simulink library "GOcontroll_Crank"  (R2023b)
settings: Solver=ode45  StartTime=0.0  StopTime=10.0  RelTol=1e-3  EnableMultiTasking=on
PreLoadFcn:
  | compile_crank_mex;
undefined symbols (not defined in the file or in its folder): DiscIntNeverNeededParam, missing
libraries: simulink x2
(part 1 of 2)
settings Model: Creator=HANcoder  LastModifiedBy=maud
settings Model: ModifiedHistory=|
  | la_obwlf -- Thu Sep 01 12:12:55 2016 -- Version 0.33
  | 
  | 
  | 
  | 
  | 
  | 
  | la_obwlf -- Thu Sep 01 09:23:34 2016 -- Version 0.33
  | changed the version in the Base Sample Time block
  | 
  | 
  | 
  | la_obwlf -- Tue Aug 30 15:48:17 2016 -- Version 0.33
settings SolverCC: AlgebraicLoopSolver=TrustRegion
settings DataIOCC: LimitDataPoints=on  SaveFormat=Array  SignalLoggingSaveFormat=ModelDataLogs  ReturnWorkspaceOutputs=off
settings OptimizationCC: ExpressionDepthLimit=2147483647  LifeSpan=inf
settings DebuggingCC: UnderspecifiedInitializationDetection=Classic  MergeDetectMultiDrivingBlocksExec=none  SolverPrmCheckMsg=warning  FcnCallInpInsideContextMsg=warning  UnconnectedInputMsg=warning  UnconnectedOutputMsg=warning  UnconnectedLineMsg=warning  StateNameClashWarn=warning  SFUnexpectedBacktrackingDiag=warning  SFNoUnconditionalDefaultTransitionDiag=warning  SFExecutionAtInitializationDiag=none  ArithmeticOperatorsInVariantConditions=warning
settings HardwareCC: ProdBitPerPointer=32  ProdBitPerSizeT=32  ProdBitPerPtrDiffT=32  ProdLargestAtomicFloat=None  ProdIntDivRoundTo=Undefined  ProdEndianess=Unspecified  ProdWordSize=32  ProdHWDeviceType=32-bit Generic
settings ModelReferenceCC: EnableRefExpFcnMdlSchedulingChecks=on  PropagateSignalLabelsOutOfModel=off
settings SFSimCC: SimUseLocalCustomCode=off  CustomCodeUndefinedFunction=UseInterfaceOnly
settings RTWCC: RTWUseLocalCustomCode=off
settings CodeAppCC: StateflowObjectComments=on
settings GRTTargetCC: TargetLangStandard=C89/C90 (ANSI)  CombineOutputUpdateFcns=off  GRTInterface=on
settings ConfigComp: CovMetricSettings=dw  CovSaveCumulativeToWorkspaceVar=on  CovSaveSingleToWorkspaceVar=on  CovExternalEMLEnable=off  CovSFcnEnable=off

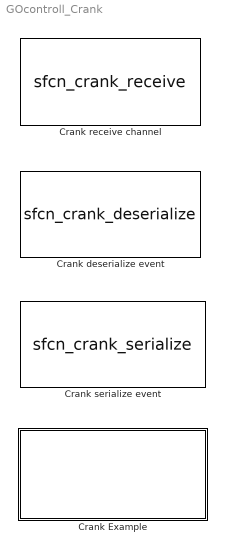
== system GOcontroll_Crank ==
  Crank Example : Subsystem
  Crank deserialize event : S-Function  FunctionName=sfcn_crank_deserialize  Parameters=channel,event_num,event_name,output_names,output_datatypes  SFunctionDeploymentMode=off  EnableBusSupport=off  mask(Crank deserialize event){channel="", event_name=event, event_num="", output_names=[], output_datatypes=[]}
      mask prompts: event_name "Event to deserialize"
      mask help:
      | Block to deserialize an event coming from a gre_io channel
      |
      | Place this block in a function call subsystem that is called by a Crank receive channel block, then link the event ports of these to blocks.
      | Multiple of this blocks can then be placed in this subsystem and attached to the event line.
      |
      | Select the event from the list to deserialize.
      mask Callback channel:
      | try
      |         graph = sltrace(gcb,"Source",TraceAll="on",BlockPath="on");
      |     catch
      |         return;
      |     end
      |     if isempty(graph.SrcBlocks)
      |         error("Could not find a source Crank receive channel block attached to this one");
      |     end
      |     receive = getBlock(graph.SrcBlocks(1),1);
      |     mask = Simulink.Mask.get(gcb);
      |     pars = mask.Parameters;
      |     set_param(gcb, 'channel', char(get_param(receive,'channel')));
      |     mask.getParameter('event_name').TypeOptions = eval(string(get_param(receive,'events')));
      mask TypeOptions event_name: event
      mask Callback event_name:
      | try
      |         graph = sltrace(gcb,"Source",TraceAll="on",BlockPath="on");
      |     catch
      |         return;
      |     end
      |     if isempty(graph.SrcBlocks)
      |         error("Could not find a source Crank receive channel block attached to this one");
      |     end
      |     receive = getBlock(graph.SrcBlocks(1),1);
      |     mask = Simulink.Mask.get(gcb);
      |     pars = mask.Parameters;
      |     set_param(gcb, 'channel', char(get_param(receive,'channel')));
      |     mask.getParameter('event_name').TypeOptions = eval(string(get_param(receive,'events')));
      |     events = eval(string(get_param(receive, 'events')));
      |     eventname = string(get_param(gcb,'event_name'));
      |     index =  find(strcmp(events,eventname));
      |     set_param(gcb, 'event_num',num2str(max(index-1, 0)));
      |     num_fields = eval(string(get_param(receive, 'num_fields')));
      |     field_types = eval(string(get_param(receive, 'field_types')));
      |     field_names = eval(string(get_param(receive, 'field_names')));
      |     if num_fields(index) > 0
      |         names = sprintf('\"%s\",',field_names(index,1:num_fields(index)));
      |         names = names(1:end-1);
      |         names = sprintf('[%s]',names);
      |         set_param(gcb, 'output_names', names);
      |         set_param(gcb, 'output_datatypes', mat2str(field_types(index,1:num_fields(index))));
      |     else
      |         set_param(gcb, 'output_names', '[]');
      |         set_param(gcb, 'output_datatypes', '[]');
      |     end
      mask Display:
      | fprintf('Crank deserialize event\n%s',event_name);
      | text(2, 6, blockset_crank_version());
      | port_label('input', 1, 'event');
      | port_label('output', 1, 'function call');
      | outputnamesarr = eval(output_names);
      | for idx = 1:length(outputnamesarr)
      |     port_label('output', idx+1, outputnamesarr(idx));
      | end
  Crank receive channel : S-Function  FunctionName=sfcn_crank_receive  Parameters=tsamp,nbuff_len,channel,events,num_events,header  SFunctionDeploymentMode=off  EnableBusSupport=off  mask(Crank receive channel){field_names=string([]), num_fields=double([]), field_types=double([]), fmts=string([]), tsamp=-1, nbuff_len=1, channel='channel', header_text=, events=string([]), header="", num_events=0}
      mask prompts: tsamp "Sample time"; nbuff_len "Crank serialized data buffer size"; channel "Crank channel name"; header_text "Header file"
      mask help:
      | Block to receive events coming through a gre_io channel
      |
      | Press the button to Select a crank header that contains the definitions of all the events on this channel.
      | Set the desired sample time to determine how often to process events
      | Set the buffer size for your gre_io_serialized_data_t buffer
      | Set the receive channel name
      mask init:
      | if ~ischar(channel)
      |         error("The channel name needs to be of type char, enter it between single quotes instead of double ones");
      |     end
      |     if nbuff_len <= 0 || mod(nbuff_len,1) > 0
      |         error("The nbuffer length needs to be a positive integer");
      |     end
      mask DialogControl Control2 Prompt: Select crank header
      mask DialogControl Control2 Callback:
      | mask = Simulink.Mask.get(gcb);
      |     pars = mask.Parameters;
      |     [file, location] = uigetfile('*.h','Get crank header');
      |     if exist(fullfile(location, file), 'file') == 2
      |         header_text = fileread(fullfile(location, file));
      |         events = processCrankHeader(header_text);
      |         set_param(gcb, 'header_text', header_text);
      |         set_param(gcb, 'header', char(sprintf("\'%s\'",file)));
      |         names = sprintf('\"%s\",',events.names);
      |         names = names(1:end-1);
      |         names = sprintf('[%s]',names);
      |         set_param(gcb, 'events', names);
      |         set_param(gcb, 'fmts', mat2str(events.fmts));
      |         set_param(gcb, 'num_fields', mat2str(events.num_fields));
      |         set_param(gcb, 'field_names', mat2str(events.field_names));
      |         set_param(gcb, 'field_types', mat2str(events.field_types));
      |         set_param(gcb, 'num_events', num2str(length(events.names)));
      |     end
      mask Display:
      | fprintf('Crank receive channel\n%s',channel);
      | text(2, 6, blockset_crank_version());
      | port_label('output', 1, 'function call');
      | port_label('output', 2, 'event');
  Crank serialize event : S-Function  FunctionName=sfcn_crank_serialize  Parameters=tsamp,channel,event_name,input_names,input_datatypes,header  SFunctionDeploymentMode=off  EnableBusSupport=off  mask(Crank serialize event){field_types=[], tsamp=-1, channel='channel', event_name=event, input_names=[], input_datatypes=[], header='', header_text=, num_fields=[], field_names=[], fmts=[], events=[]}
      mask prompts: tsamp "Sample time"; channel "Crank channel name"; event_name "Event to serialize"; header_text "Header file"
      mask help:
      | Block to serialize an event and send it through a gre_io channel
      |
      | Set the sample time to set the update rate of the display
      | Set the channel name on which the events are sent
      | Press the button to select a crank header that contains the event definitions
      | Select an event from the now loaded event list
      mask init:
      | if ~ischar(channel)
      |         error("The channel name needs to be of type char, enter it between single quotes instead of double ones");
      |     end
      mask TypeOptions event_name: event
      mask Callback event_name:
      | events = eval(string(get_param(gcb, 'events')));
      |     eventname = char(get_param(gcb,'event_name'));
      |     index =  find(strcmp(events,eventname));
      |     num_fields = eval(string(get_param(gcb, 'num_fields')));
      |     field_types = eval(string(get_param(gcb, 'field_types')));
      |     field_names = eval(string(get_param(gcb, 'field_names')));
      |     if num_fields(index) > 0
      |         names = sprintf('\"%s\",',field_names(index,1:num_fields(index)));
      |         names = names(1:end-1);
      |         names = sprintf('[%s]',names);
      |         set_param(gcb, 'input_names', names);
      |         set_param(gcb, 'input_datatypes', mat2str(field_types(index,1:num_fields(index))));
      |     else
      |         set_param(gcb, 'input_names', '[]');
      |         set_param(gcb, 'input_datatypes', '[]');
      |     end
      mask DialogControl Control2 Prompt: Select crank header
      mask DialogControl Control2 Callback:
      | mask = Simulink.Mask.get(gcb);
      |     pars = mask.Parameters;
      |     [file, location] = uigetfile('*.h','Get crank header');
      |     if exist(fullfile(location, file), 'file') == 2
      |         header_text = fileread(fullfile(location, file));
      |         events = processCrankHeader(header_text);
      |         set_param(gcb, 'header_text', header_text);
      |         set_param(gcb, 'header', char(sprintf("\'%s\'",file)));
      |         mask.getParameter('event_name').TypeOptions = events.names;
      |         set_param(gcb, 'events', mat2str(events.names));
      |         set_param(gcb, 'fmts', mat2str(events.fmts));
      |         set_param(gcb, 'num_fields', mat2str(events.num_fields));
      |         set_param(gcb, 'field_names', mat2str(events.field_names));
      |         set_param(gcb, 'field_types', mat2str(events.field_types));
      |     end
      mask Display:
      | fprintf('Crank serialize event\nChannel: %s\nEvent: %s',channel, event_name);
      | text(2, 6, blockset_crank_version());
      | inputnamesarr = eval(input_names);
      | for idx = 1:length(inputnamesarr)
      |     port_label('input', idx, inputnamesarr(idx));
      | end

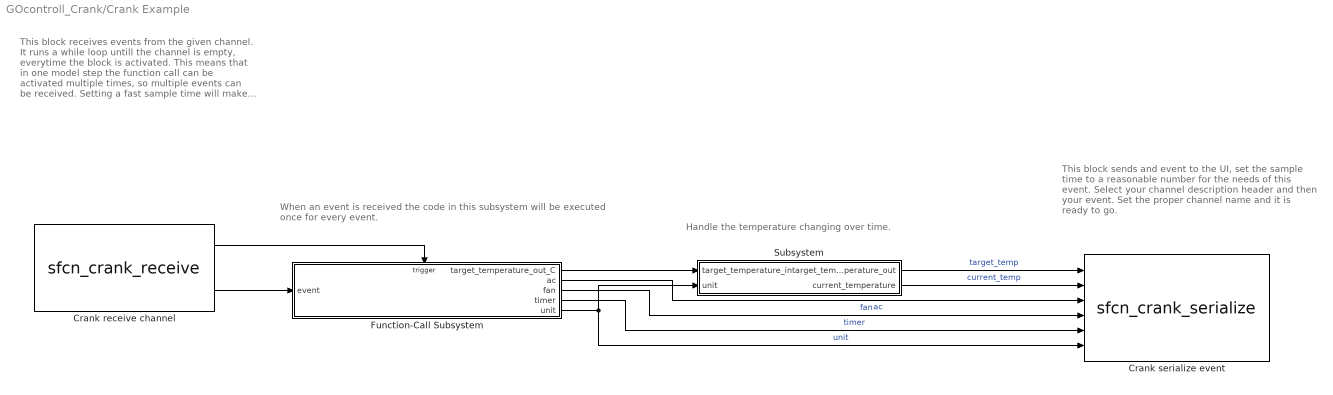
== system GOcontroll_Crank/Crank Example ==
  note: This block sends and event to the UI, set
      | the sample time to a reasonable number
      | for the needs of this event.
      | Select your channel description header
      | and then your event. Set the proper
      | channel name and it is ready to go.
  note: Handle the temperature changing over
      | time.
  note: When an event is received the code in this subsystem
      | will be executed once for every event.
  note: This block receives events from the
      | given channel. It runs a while loop
      | untill the channel is empty, everytime
      | the block is activated.
      | This means that in one model step
      | the function call can be activated
      | multiple times, so multiple events
      | can be received.
      | Setting a fast sample time will make
      | simulink read from the channel more
      | often, giving faster response times but
      | slightly more overhead, though this
      | should not be very significant.
  Crank receive channel : S-Function  AncestorBlock=GOcontroll_Crank/Crank receive channel  FunctionName=sfcn_crank_receive  Parameters=tsamp,nbuff_len,channel,events,num_events,header  SFunctionDeploymentMode=off  EnableBusSupport=off  mask(Crank receive channel){field_names=["num" "unit" string(missing) string(missing) string(missing) string(missing);"num" "unit" string(missing) string(missing) string(missing) string(missing);"target_temperature" "current_temperature" "ac" "fan" "timer" "units"], num_fields=[2 2 6 0 0 0 0], field_types=[5 5 0 0 0 0;5 5 0 0 0 0;4 4 3 3 3 3], fmts=["2u1 num 2u1 unit" "2u1 num 2u1 unit" "2s1 target_temperature 2s1 current_temperature 1u1 ac 1u1 fan 1u1 timer 1u1 units" "" "" "" ""], tsamp=0.01, nbuff_len=100, channel='thermostat_backend', header_text=|, events=["decrease_temperature","increase_temperature","thermostat_update","toggle_ac","toggle_fan","toggle_timer","toggle_units"], header='ThermostatIO_events.h', num_events=7}
      mask header_text=|
      | #define DECREASE_TEMPERATURE_EVENT "decrease_temperature"
      | #define DECREASE_TEMPERATURE_FMT "2u1 num 2u1 unit"
      | typedef struct {
      | 	uint16_t 		num;
      | 	uint16_t 		unit;
      | } decrease_temperature_event_t;
      |
      | #define INCREASE_TEMPERATURE_EVENT "increase_temperature"
      | #define INCREASE_TEMPERATURE_FMT "2u1 num 2u1 unit"
      | typedef struct {
      | 	uint16_t 		num;
      | 	uint16_t 		unit;
      | } increase_temperature_event_t;
      |
      | #define THERMOSTAT_UPDATE_EVENT "thermostat_update"
      | #define THERMOSTAT_UPDATE_FMT "2s1 target_temperature 2s1 current_temperature 1u1 ac 1u1 fan 1u1 timer 1u1 units"
      | typedef struct {
      | 	int16_t 		target_temperature;
      | 	int16_t 		current_temperature;
      | 	uint8_t 		ac;
      | 	uint8_t 		fan;
      | 	uint8_t 		timer;
      | 	uint8_t 		units;
      | } thermostat_update_event_t;
      |
      | #define TOGGLE_AC_EVENT "toggle_ac"
      |
      | #define TOGGLE_FAN_EVENT "toggle_fan"
      |
      | #define TOGGLE_TIMER_EVENT "toggle_timer"
      |
      | #define TOGGLE_UNITS_EVENT "toggle_units"
      mask prompts: tsamp "Sample time"; nbuff_len "Crank serialized data buffer size"; channel "Crank channel name"; header_text "Header file"
      mask help:
      | Block to receive events coming through a gre_io channel
      |
      | Press the button to Select a crank header that contains the definitions of all the events on this channel.
      | Set the desired sample time to determine how often to process events
      | Set the buffer size for your gre_io_serialized_data_t buffer
      | Set the receive channel name
      mask init: same as GOcontroll_Crank/Crank receive channel
      mask DialogControl Control2 Prompt: Select crank header
      mask DialogControl Control2 Callback:
      | mask = Simulink.Mask.get(gcb);
      |     pars = mask.Parameters;
      |     [file, location] = uigetfile('*.h','Get crank header');
      |     if exist(fullfile(location, file), 'file') == 2
      |         header_text = fileread(fullfile(location, file));
      |         events = processCrankHeader(header_text);
      |         set_param(gcb, 'header_text', header_text);
      |         set_param(gcb, 'header', char(sprintf("\'%s\'",file)));
      |         names = sprintf('\"%s\",',events.names);
      |         names = names(1:end-1);
      |         names = sprintf('[%s]',names);
      |         set_param(gcb, 'events', names);
      |         set_param(gcb, 'fmts', mat2str(events.fmts));
      |         set_param(gcb, 'num_fields', mat2str(events.num_fields));
      |         set_param(gcb, 'field_names', mat2str(events.field_names));
      |         set_param(gcb, 'field_types', mat2str(events.field_types));
      |         set_param(gcb, 'num_events', num2str(length(events.names)));
      |     end
      mask Display:
      | fprintf('Crank receive channel\n%s',channel);
      | text(2, 6, blockset_crank_version());
      | port_label('output', 1, 'function call');
      | port_label('output', 2, 'event');
  Crank serialize event : S-Function  AncestorBlock=GOcontroll_Crank/Crank serialize event  FunctionName=sfcn_crank_serialize  Parameters=tsamp,channel,event_name,input_names,input_datatypes,header  SFunctionDeploymentMode=off  EnableBusSupport=off  mask(Crank serialize event){field_types=[5 5 0 0 0 0;5 5 0 0 0 0;4 4 3 3 3 3], tsamp=0.02, channel='thermostat_frontend', event_name=thermostat_update, input_names=["target_temperature","current_temperature","ac","fan","timer","units"], input_datatypes=[4 4 3 3 3 3], header='ThermostatIO_events.h', header_text=|, num_fields=[2 2 6 0 0 0 0], field_names=["num" "unit" string(missing) string(missing) string(missing) string(missing);"num" "unit" string(missing) string(missing) string(missing) string(missing);"target_temperature" "current_temperature" "ac" "fan" "timer" "units"], fmts=["2u1 num 2u1 unit" "2u1 num 2u1 unit" "2s1 target_temperature 2s1 current_temperature 1u1 ac 1u1 fan 1u1 timer 1u1 units" "" "" "" ""], events=["decrease_temperature" "increase_temperature" "thermostat_update" "toggle_ac" "toggle_fan" "toggle_timer" "toggle_units"]}
      mask header_text=|
      | #define DECREASE_TEMPERATURE_EVENT "decrease_temperature"
      | #define DECREASE_TEMPERATURE_FMT "2u1 num 2u1 unit"
      | typedef struct {
      | 	uint16_t 		num;
      | 	uint16_t 		unit;
      | } decrease_temperature_event_t;
      |
      | #define INCREASE_TEMPERATURE_EVENT "increase_temperature"
      | #define INCREASE_TEMPERATURE_FMT "2u1 num 2u1 unit"
      | typedef struct {
      | 	uint16_t 		num;
      | 	uint16_t 		unit;
      | } increase_temperature_event_t;
      |
      | #define THERMOSTAT_UPDATE_EVENT "thermostat_update"
      | #define THERMOSTAT_UPDATE_FMT "2s1 target_temperature 2s1 current_temperature 1u1 ac 1u1 fan 1u1 timer 1u1 units"
      | typedef struct {
      | 	int16_t 		target_temperature;
      | 	int16_t 		current_temperature;
      | 	uint8_t 		ac;
      | 	uint8_t 		fan;
      | 	uint8_t 		timer;
      | 	uint8_t 		units;
      | } thermostat_update_event_t;
      |
      | #define TOGGLE_AC_EVENT "toggle_ac"
      |
      | #define TOGGLE_FAN_EVENT "toggle_fan"
      |
      | #define TOGGLE_TIMER_EVENT "toggle_timer"
      |
      | #define TOGGLE_UNITS_EVENT "toggle_units"
      mask prompts: tsamp "Sample time"; channel "Crank channel name"; event_name "Event to serialize"; header_text "Header file"
      mask help:
      | Block to serialize an event and send it through a gre_io channel
      |
      | Set the sample time to set the update rate of the display
      | Set the channel name on which the events are sent
      | Press the button to select a crank header that contains the event definitions
      | Select an event from the now loaded event list
      mask init:
      | if ~ischar(channel)
      |         error("The channel name needs to be of type char, enter it between single quotes instead of double ones");
      |     end
      mask TypeOptions event_name: event
      mask Callback event_name:
      | events = eval(string(get_param(gcb, 'events')));
      |     eventname = char(get_param(gcb,'event_name'));
      |     index =  find(strcmp(events,eventname));
      |     num_fields = eval(string(get_param(gcb, 'num_fields')));
      |     field_types = eval(string(get_param(gcb, 'field_types')));
      |     field_names = eval(string(get_param(gcb, 'field_names')));
      |     if num_fields(index) > 0
      |         names = sprintf('\"%s\",',field_names(index,1:num_fields(index)));
      |         names = names(1:end-1);
      |         names = sprintf('[%s]',names);
      |         set_param(gcb, 'input_names', names);
      |         set_param(gcb, 'input_datatypes', mat2str(field_types(index,1:num_fields(index))));
      |     else
      |         set_param(gcb, 'input_names', '[]');
      |         set_param(gcb, 'input_datatypes', '[]');
      |     end
      mask DialogControl Control2 Prompt: Select crank header
      mask DialogControl Control2 Callback:
      | mask = Simulink.Mask.get(gcb);
      |     pars = mask.Parameters;
      |     [file, location] = uigetfile('*.h','Get crank header');
      |     if exist(fullfile(location, file), 'file') == 2
      |         header_text = fileread(fullfile(location, file));
      |         events = processCrankHeader(header_text);
      |         set_param(gcb, 'header_text', header_text);
      |         set_param(gcb, 'header', char(sprintf("\'%s\'",file)));
      |         mask.getParameter('event_name').TypeOptions = events.names;
      |         set_param(gcb, 'events', mat2str(events.names));
      |         set_param(gcb, 'fmts', mat2str(events.fmts));
      |         set_param(gcb, 'num_fields', mat2str(events.num_fields));
      |         set_param(gcb, 'field_names', mat2str(events.field_names));
      |         set_param(gcb, 'field_types', mat2str(events.field_types));
      |     end
      mask Display:
      | fprintf('Crank serialize event\nChannel: %s\nEvent: %s',channel, event_name);
      | text(2, 6, blockset_crank_version());
      | inputnamesarr = eval(input_names);
      | for idx = 1:length(inputnamesarr)
      |     port_label('input', idx, inputnamesarr(idx));
      | end
  Function-Call Subsystem : Subsystem  TreatAsAtomicUnit=on
  Subsystem : Subsystem
  wires:
  Subsystem/1(target_temperature_out) -> Crank serialize event/1  "target_temp"
  Function-Call Subsystem/1(target_temperature_out_C) -> Subsystem/1(target_temperature_in)
  Subsystem/2(current_temperature) -> Crank serialize event/2  "current_temp"
  Function-Call Subsystem/5(unit) -> Crank serialize event/6, Subsystem/2(unit)  "unit"
  Function-Call Subsystem/4(timer) -> Crank serialize event/5  "timer"
  Function-Call Subsystem/3(fan) -> Crank serialize event/4  "fan"
  Function-Call Subsystem/2(ac) -> Crank serialize event/3  "ac"
  Crank receive channel/2 -> Function-Call Subsystem/1(event)
  Crank receive channel/1 -> Function-Call Subsystem/Trigger

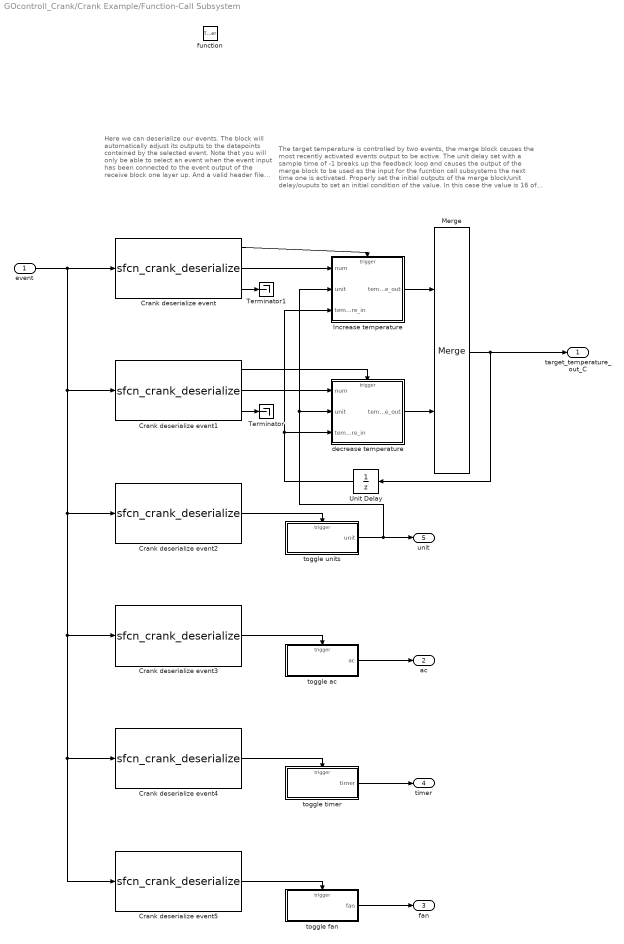
== system GOcontroll_Crank/Crank Example/Function-Call Subsystem ==
  note: The target temperature is controlled by two events, the merge
      | block causes the most recently activated events output to be
      | active. The unit delay set with a sample time of -1 breaks up
      | the feedback loop and causes the output of the merge block
      | to be used as the input for the fucntion call subsystems the
      | next time one is activated. Properly set the initial outputs of
      | the merge block/unit delay/ouputs to set an initial condition of
      | the value. In this case the value is 16 of datatype single.
  note: Here we can deserialize our events.
      | The block will automatically adjust its
      | outputs to the datapoints contained by
      | the selected event.
      | Note that you will only be able to select
      | an event when the event input has
      | been connected to the event output of
      | the receive block one layer up. And a
      | valid header file has been select there.
  event : Inport
  function : TriggerPort  TriggerType=function-call  VariantControl=(inherit)
  Crank deserialize event : S-Function  AncestorBlock=GOcontroll_Crank/Crank deserialize event  FunctionName=sfcn_crank_deserialize  Parameters=channel,event_num,event_name,output_names,output_datatypes  SFunctionDeploymentMode=off  EnableBusSupport=off  mask(Crank deserialize event){channel='thermostat_backend', event_name=increase_temperature, event_num=1, output_names=["num","unit"], output_datatypes=[5 5]}
      mask prompts: event_name "Event to deserialize"
      mask help:
      | Block to deserialize an event coming from a gre_io channel
      |
      | Place this block in a function call subsystem that is called by a Crank receive channel block, then link the event ports of these to blocks.
      | Multiple of this blocks can then be placed in this subsystem and attached to the event line.
      |
      | Select the event from the list to deserialize.
      mask Callback channel:
      | try
      |         graph = sltrace(gcb,"Source",TraceAll="on",BlockPath="on");
      |     catch
      |         return;
      |     end
      |     if isempty(graph.SrcBlocks)
      |         error("Could not find a source Crank receive channel block attached to this one");
      |     end
      |     receive = getBlock(graph.SrcBlocks(1),1);
      |     mask = Simulink.Mask.get(gcb);
      |     pars = mask.Parameters;
      |     set_param(gcb, 'channel', char(get_param(receive,'channel')));
      |     mask.getParameter('event_name').TypeOptions = eval(string(get_param(receive,'events')));
      mask TypeOptions event_name: decrease_temperature | increase_temperature | thermostat_update | toggle_ac | toggle_fan | toggle_timer | toggle_units
      mask Callback event_name:
      | try
      |         graph = sltrace(gcb,"Source",TraceAll="on",BlockPath="on");
      |     catch
      |         return;
      |     end
      |     if isempty(graph.SrcBlocks)
      |         error("Could not find a source Crank receive channel block attached to this one");
      |     end
      |     receive = getBlock(graph.SrcBlocks(1),1);
      |     mask = Simulink.Mask.get(gcb);
      |     pars = mask.Parameters;
      |     set_param(gcb, 'channel', char(get_param(receive,'channel')));
      |     mask.getParameter('event_name').TypeOptions = eval(string(get_param(receive,'events')));
      |     events = eval(string(get_param(receive, 'events')));
      |     eventname = string(get_param(gcb,'event_name'));
      |     index =  find(strcmp(events,eventname));
      |     set_param(gcb, 'event_num',num2str(max(index-1, 0)));
      |     num_fields = eval(string(get_param(receive, 'num_fields')));
      |     field_types = eval(string(get_param(receive, 'field_types')));
      |     field_names = eval(string(get_param(receive, 'field_names')));
      |     if num_fields(index) > 0
      |         names = sprintf('\"%s\",',field_names(index,1:num_fields(index)));
      |         names = names(1:end-1);
      |         names = sprintf('[%s]',names);
      |         set_param(gcb, 'output_names', names);
      |         set_param(gcb, 'output_datatypes', mat2str(field_types(index,1:num_fields(index))));
      |     else
      |         set_param(gcb, 'output_names', '[]');
      |         set_param(gcb, 'output_datatypes', '[]');
      |     end
      mask Display:
      | fprintf('Crank deserialize event\n%s',event_name);
      | text(2, 6, blockset_crank_version());
      | port_label('input', 1, 'event');
      | port_label('output', 1, 'function call');
      | outputnamesarr = eval(output_names);
      | for idx = 1:length(outputnamesarr)
      |     port_label('output', idx+1, outputnamesarr(idx));
      | end
  Crank deserialize event1 : S-Function  AncestorBlock=GOcontroll_Crank/Crank deserialize event  FunctionName=sfcn_crank_deserialize  Parameters=channel,event_num,event_name,output_names,output_datatypes  SFunctionDeploymentMode=off  EnableBusSupport=off  mask(Crank deserialize event){channel='thermostat_backend', event_name=decrease_temperature, event_num=0, output_names=["num","unit"], output_datatypes=[5 5]}
      mask prompts: event_name "Event to deserialize"
      mask help:
      | Block to deserialize an event coming from a gre_io channel
      |
      | Place this block in a function call subsystem that is called by a Crank receive channel block, then link the event ports of these to blocks.
      | Multiple of this blocks can then be placed in this subsystem and attached to the event line.
      |
      | Select the event from the list to deserialize.
      mask Callback channel:
      | try
      |         graph = sltrace(gcb,"Source",TraceAll="on",BlockPath="on");
      |     catch
      |         return;
      |     end
      |     if isempty(graph.SrcBlocks)
      |         error("Could not find a source Crank receive channel block attached to this one");
      |     end
      |     receive = getBlock(graph.SrcBlocks(1),1);
      |     mask = Simulink.Mask.get(gcb);
      |     pars = mask.Parameters;
      |     set_param(gcb, 'channel', char(get_param(receive,'channel')));
      |     mask.getParameter('event_name').TypeOptions = eval(string(get_param(receive,'events')));
      mask TypeOptions event_name: decrease_temperature | increase_temperature | thermostat_update | toggle_ac | toggle_fan | toggle_timer | toggle_units
      mask Callback event_name:
      | try
      |         graph = sltrace(gcb,"Source",TraceAll="on",BlockPath="on");
      |     catch
      |         return;
      |     end
      |     if isempty(graph.SrcBlocks)
      |         error("Could not find a source Crank receive channel block attached to this one");
      |     end
      |     receive = getBlock(graph.SrcBlocks(1),1);
      |     mask = Simulink.Mask.get(gcb);
      |     pars = mask.Parameters;
      |     set_param(gcb, 'channel', char(get_param(receive,'channel')));
      |     mask.getParameter('event_name').TypeOptions = eval(string(get_param(receive,'events')));
      |     events = eval(string(get_param(receive, 'events')));
      |     eventname = string(get_param(gcb,'event_name'));
      |     index =  find(strcmp(events,eventname));
      |     set_param(gcb, 'event_num',num2str(max(index-1, 0)));
      |     num_fields = eval(string(get_param(receive, 'num_fields')));
      |     field_types = eval(string(get_param(receive, 'field_types')));
      |     field_names = eval(string(get_param(receive, 'field_names')));
      |     if num_fields(index) > 0
      |         names = sprintf('\"%s\",',field_names(index,1:num_fields(index)));
      |         names = names(1:end-1);
      |         names = sprintf('[%s]',names);
      |         set_param(gcb, 'output_names', names);
      |         set_param(gcb, 'output_datatypes', mat2str(field_types(index,1:num_fields(index))));
      |     else
      |         set_param(gcb, 'output_names', '[]');
      |         set_param(gcb, 'output_datatypes', '[]');
      |     end
      mask Display:
      | fprintf('Crank deserialize event\n%s',event_name);
      | text(2, 6, blockset_crank_version());
      | port_label('input', 1, 'event');
      | port_label('output', 1, 'function call');
      | outputnamesarr = eval(output_names);
      | for idx = 1:length(outputnamesarr)
      |     port_label('output', idx+1, outputnamesarr(idx));
      | end
  Crank deserialize event2 : S-Function  AncestorBlock=GOcontroll_Crank/Crank deserialize event  FunctionName=sfcn_crank_deserialize  Parameters=channel,event_num,event_name,output_names,output_datatypes  SFunctionDeploymentMode=off  EnableBusSupport=off  mask(Crank deserialize event){channel='thermostat_backend', event_name=toggle_units, event_num=6, output_names=[], output_datatypes=[]}
      mask prompts: event_name "Event to deserialize"
      mask help:
      | Block to deserialize an event coming from a gre_io channel
      |
      | Place this block in a function call subsystem that is called by a Crank receive channel block, then link the event ports of these to blocks.
      | Multiple of this blocks can then be placed in this subsystem and attached to the event line.
      |
      | Select the event from the list to deserialize.
      mask Callback channel:
      | try
      |         graph = sltrace(gcb,"Source",TraceAll="on",BlockPath="on");
      |     catch
      |         return;
      |     end
      |     if isempty(graph.SrcBlocks)
      |         error("Could not find a source Crank receive channel block attached to this one");
      |     end
      |     receive = getBlock(graph.SrcBlocks(1),1);
      |     mask = Simulink.Mask.get(gcb);
      |     pars = mask.Parameters;
      |     set_param(gcb, 'channel', char(get_param(receive,'channel')));
      |     mask.getParameter('event_name').TypeOptions = eval(string(get_param(receive,'events')));
      mask TypeOptions event_name: decrease_temperature | increase_temperature | thermostat_update | toggle_ac | toggle_fan | toggle_timer | toggle_units
      mask Callback event_name:
      | try
      |         graph = sltrace(gcb,"Source",TraceAll="on",BlockPath="on");
      |     catch
      |         return;
      |     end
      |     if isempty(graph.SrcBlocks)
      |         error("Could not find a source Crank receive channel block attached to this one");
      |     end
      |     receive = getBlock(graph.SrcBlocks(1),1);
      |     mask = Simulink.Mask.get(gcb);
      |     pars = mask.Parameters;
      |     set_param(gcb, 'channel', char(get_param(receive,'channel')));
      |     mask.getParameter('event_name').TypeOptions = eval(string(get_param(receive,'events')));
      |     events = eval(string(get_param(receive, 'events')));
      |     eventname = string(get_param(gcb,'event_name'));
      |     index =  find(strcmp(events,eventname));
      |     set_param(gcb, 'event_num',num2str(max(index-1, 0)));
      |     num_fields = eval(string(get_param(receive, 'num_fields')));
      |     field_types = eval(string(get_param(receive, 'field_types')));
      |     field_names = eval(string(get_param(receive, 'field_names')));
      |     if num_fields(index) > 0
      |         names = sprintf('\"%s\",',field_names(index,1:num_fields(index)));
      |         names = names(1:end-1);
      |         names = sprintf('[%s]',names);
      |         set_param(gcb, 'output_names', names);
      |         set_param(gcb, 'output_datatypes', mat2str(field_types(index,1:num_fields(index))));
      |     else
      |         set_param(gcb, 'output_names', '[]');
      |         set_param(gcb, 'output_datatypes', '[]');
      |     end
      mask Display:
      | fprintf('Crank deserialize event\n%s',event_name);
      | text(2, 6, blockset_crank_version());
      | port_label('input', 1, 'event');
      | port_label('output', 1, 'function call');
      | outputnamesarr = eval(output_names);
      | for idx = 1:length(outputnamesarr)
      |     port_label('output', idx+1, outputnamesarr(idx));
      | end
  Crank deserialize event3 : S-Function  AncestorBlock=GOcontroll_Crank/Crank deserialize event  FunctionName=sfcn_crank_deserialize  Parameters=channel,event_num,event_name,output_names,output_datatypes  SFunctionDeploymentMode=off  EnableBusSupport=off  mask(Crank deserialize event){channel='thermostat_backend', event_name=toggle_ac, event_num=3, output_names=[], output_datatypes=[]}
      mask prompts: event_name "Event to deserialize"
      mask help:
      | Block to deserialize an event coming from a gre_io channel
      |
      | Place this block in a function call subsystem that is called by a Crank receive channel block, then link the event ports of these to blocks.
      | Multiple of this blocks can then be placed in this subsystem and attached to the event line.
      |
      | Select the event from the list to deserialize.
      mask Callback channel:
      | try
      |         graph = sltrace(gcb,"Source",TraceAll="on",BlockPath="on");
      |     catch
      |         return;
      |     end
      |     if isempty(graph.SrcBlocks)
      |         error("Could not find a source Crank receive channel block attached to this one");
      |     end
      |     receive = getBlock(graph.SrcBlocks(1),1);
      |     mask = Simulink.Mask.get(gcb);
      |     pars = mask.Parameters;
      |     set_param(gcb, 'channel', char(get_param(receive,'channel')));
      |     mask.getParameter('event_name').TypeOptions = eval(string(get_param(receive,'events')));
      mask TypeOptions event_name: decrease_temperature | increase_temperature | thermostat_update | toggle_ac | toggle_fan | toggle_timer | toggle_units
      mask Callback event_name:
      | try
      |         graph = sltrace(gcb,"Source",TraceAll="on",BlockPath="on");
      |     catch
      |         return;
      |     end
      |     if isempty(graph.SrcBlocks)
      |         error("Could not find a source Crank receive channel block attached to this one");
      |     end
      |     receive = getBlock(graph.SrcBlocks(1),1);
      |     mask = Simulink.Mask.get(gcb);
      |     pars = mask.Parameters;
      |     set_param(gcb, 'channel', char(get_param(receive,'channel')));
      |     mask.getParameter('event_name').TypeOptions = eval(string(get_param(receive,'events')));
      |     events = eval(string(get_param(receive, 'events')));
      |     eventname = string(get_param(gcb,'event_name'));
      |     index =  find(strcmp(events,eventname));
      |     set_param(gcb, 'event_num',num2str(max(index-1, 0)));
      |     num_fields = eval(string(get_param(receive, 'num_fields')));
      |     field_types = eval(string(get_param(receive, 'field_types')));
      |     field_names = eval(string(get_param(receive, 'field_names')));
      |     if num_fields(index) > 0
      |         names = sprintf('\"%s\",',field_names(index,1:num_fields(index)));
      |         names = names(1:end-1);
      |         names = sprintf('[%s]',names);
      |         set_param(gcb, 'output_names', names);
      |         set_param(gcb, 'output_datatypes', mat2str(field_types(index,1:num_fields(index))));
      |     else
      |         set_param(gcb, 'output_names', '[]');
      |         set_param(gcb, 'output_datatypes', '[]');
      |     end
      mask Display:
      | fprintf('Crank deserialize event\n%s',event_name);
      | text(2, 6, blockset_crank_version());
      | port_label('input', 1, 'event');
      | port_label('output', 1, 'function call');
      | outputnamesarr = eval(output_names);
      | for idx = 1:length(outputnamesarr)
      |     port_label('output', idx+1, outputnamesarr(idx));
      | end
  Crank deserialize event4 : S-Function  AncestorBlock=GOcontroll_Crank/Crank deserialize event  FunctionName=sfcn_crank_deserialize  Parameters=channel,event_num,event_name,output_names,output_datatypes  SFunctionDeploymentMode=off  EnableBusSupport=off  mask(Crank deserialize event){channel='thermostat_backend', event_name=toggle_timer, event_num=5, output_names=[], output_datatypes=[]}
      mask prompts: event_name "Event to deserialize"
      mask help:
      | Block to deserialize an event coming from a gre_io channel
      |
      | Place this block in a function call subsystem that is called by a Crank receive channel block, then link the event ports of these to blocks.
      | Multiple of this blocks can then be placed in this subsystem and attached to the event line.
      |
      | Select the event from the list to deserialize.
      mask Callback channel:
      | try
      |         graph = sltrace(gcb,"Source",TraceAll="on",BlockPath="on");
      |     catch
      |         return;
      |     end
      |     if isempty(graph.SrcBlocks)
      |         error("Could not find a source Crank receive channel block attached to this one");
      |     end
      |     receive = getBlock(graph.SrcBlocks(1),1);
      |     mask = Simulink.Mask.get(gcb);
      |     pars = mask.Parameters;
      |     set_param(gcb, 'channel', char(get_param(receive,'channel')));
      |     mask.getParameter('event_name').TypeOptions = eval(string(get_param(receive,'events')));
      mask TypeOptions event_name: decrease_temperature | increase_temperature | thermostat_update | toggle_ac | toggle_fan | toggle_timer | toggle_units
      mask Callback event_name:
      | try
      |         graph = sltrace(gcb,"Source",TraceAll="on",BlockPath="on");
      |     catch
      |         return;
      |     end
      |     if isempty(graph.SrcBlocks)
      |         error("Could not find a source Crank receive channel block attached to this one");
      |     end
      |     receive = getBlock(graph.SrcBlocks(1),1);
      |     mask = Simulink.Mask.get(gcb);
      |     pars = mask.Parameters;
      |     set_param(gcb, 'channel', char(get_param(receive,'channel')));
      |     mask.getParameter('event_name').TypeOptions = eval(string(get_param(receive,'events')));
      |     events = eval(string(get_param(receive, 'events')));
      |     eventname = string(get_param(gcb,'event_name'));
      |     index =  find(strcmp(events,eventname));
      |     set_param(gcb, 'event_num',num2str(max(index-1, 0)));
      |     num_fields = eval(string(get_param(receive, 'num_fields')));
      |     field_types = eval(string(get_param(receive, 'field_types')));
      |     field_names = eval(string(get_param(receive, 'field_names')));
      |     if num_fields(index) > 0
      |         names = sprintf('\"%s\",',field_names(index,1:num_fields(index)));
      |         names = names(1:end-1);
      |         names = sprintf('[%s]',names);
      |         set_param(gcb, 'output_names', names);
      |         set_param(gcb, 'output_datatypes', mat2str(field_types(index,1:num_fields(index))));
      |     else
      |         set_param(gcb, 'output_names', '[]');
      |         set_param(gcb, 'output_datatypes', '[]');
      |     end
      mask Display:
      | fprintf('Crank deserialize event\n%s',event_name);
      | text(2, 6, blockset_crank_version());
      | port_label('input', 1, 'event');
      | port_label('output', 1, 'function call');
      | outputnamesarr = eval(output_names);
      | for idx = 1:length(outputnamesarr)
      |     port_label('output', idx+1, outputnamesarr(idx));
      | end
  Crank deserialize event5 : S-Function  AncestorBlock=GOcontroll_Crank/Crank deserialize event  FunctionName=sfcn_crank_deserialize  Parameters=channel,event_num,event_name,output_names,output_datatypes  SFunctionDeploymentMode=off  EnableBusSupport=off  mask(Crank deserialize event){channel='thermostat_backend', event_name=toggle_fan, event_num=4, output_names=[], output_datatypes=[]}
      mask prompts: event_name "Event to deserialize"
      mask help:
      | Block to deserialize an event coming from a gre_io channel
      |
      | Place this block in a function call subsystem that is called by a Crank receive channel block, then link the event ports of these to blocks.
      | Multiple of this blocks can then be placed in this subsystem and attached to the event line.
      |
      | Select the event from the list to deserialize.
      mask Callback channel:
      | try
      |         graph = sltrace(gcb,"Source",TraceAll="on",BlockPath="on");
      |     catch
      |         return;
      |     end
      |     if isempty(graph.SrcBlocks)
      |         error("Could not find a source Crank receive channel block attached to this one");
      |     end
      |     receive = getBlock(graph.SrcBlocks(1),1);
      |     mask = Simulink.Mask.get(gcb);
      |     pars = mask.Parameters;
      |     set_param(gcb, 'channel', char(get_param(receive,'channel')));
      |     mask.getParameter('event_name').TypeOptions = eval(string(get_param(receive,'events')));
      mask TypeOptions event_name: decrease_temperature | increase_temperature | thermostat_update | toggle_ac | toggle_fan | toggle_timer | toggle_units
      mask Callback event_name:
      | try
      |         graph = sltrace(gcb,"Source",TraceAll="on",BlockPath="on");
      |     catch
      |         return;
      |     end
      |     if isempty(graph.SrcBlocks)
      |         error("Could not find a source Crank receive channel block attached to this one");
      |     end
      |     receive = getBlock(graph.SrcBlocks(1),1);
      |     mask = Simulink.Mask.get(gcb);
      |     pars = mask.Parameters;
      |     set_param(gcb, 'channel', char(get_param(receive,'channel')));
      |     mask.getParameter('event_name').TypeOptions = eval(string(get_param(receive,'events')));
      |     events = eval(string(get_param(receive, 'events')));
      |     eventname = string(get_param(gcb,'event_name'));
      |     index =  find(strcmp(events,eventname));
      |     set_param(gcb, 'event_num',num2str(max(index-1, 0)));
      |     num_fields = eval(string(get_param(receive, 'num_fields')));
      |     field_types = eval(string(get_param(receive, 'field_types')));
      |     field_names = eval(string(get_param(receive, 'field_names')));
      |     if num_fields(index) > 0
      |         names = sprintf('\"%s\",',field_names(index,1:num_fields(index)));
      |         names = names(1:end-1);
      |         names = sprintf('[%s]',names);
      |         set_param(gcb, 'output_names', names);
      |         set_param(gcb, 'output_datatypes', mat2str(field_types(index,1:num_fields(index))));
      |     else
      |         set_param(gcb, 'output_names', '[]');
      |         set_param(gcb, 'output_datatypes', '[]');
      |     end
      mask Display:
      | fprintf('Crank deserialize event\n%s',event_name);
      | text(2, 6, blockset_crank_version());
      | port_label('input', 1, 'event');
      | port_label('output', 1, 'function call');
      | outputnamesarr = eval(output_names);
      | for idx = 1:length(outputnamesarr)
      |     port_label('output', idx+1, outputnamesarr(idx));
      | end
  Increase temperature : Subsystem  TreatAsAtomicUnit=on
  Merge : Merge  InitialOutput=single(16)
  Terminator : Terminator
  Terminator1 : Terminator
  Unit Delay : UnitDelay  InitialCondition=single(16)  SampleTime=-1  HasFrameUpgradeWarning=on
  decrease temperature : Subsystem  TreatAsAtomicUnit=on
  toggle ac : Subsystem  TreatAsAtomicUnit=on
  toggle fan : Subsystem  TreatAsAtomicUnit=on
  toggle timer : Subsystem  TreatAsAtomicUnit=on
  toggle units : Subsystem  TreatAsAtomicUnit=on
  target_temperature_out_C : Outport
  ac : Outport  Port=2
  fan : Outport  Port=3
  timer : Outport  Port=4
  unit : Outport  Port=5
  wires:
  Crank deserialize event/3 -> Terminator1/1
  Crank deserialize event1/3 -> Terminator/1
  Merge/1 -> target_temperature_out_C/1, Unit Delay/1
  Unit Delay/1 -> decrease temperature/3(temperature_in), Increase temperature/3(temperature_in)
  toggle fan/1(fan) -> fan/1
  Crank deserialize event5/1 -> toggle fan/Trigger
  Crank deserialize event4/1 -> toggle timer/Trigger
  toggle timer/1(timer) -> timer/1
  toggle ac/1(ac) -> ac/1
  Crank deserialize event3/1 -> toggle ac/Trigger
  toggle units/1(unit) -> unit/1, decrease temperature/2(unit), Increase temperature/2(unit)
  Crank deserialize event2/1 -> toggle units/Trigger
  Increase temperature/1(temperature_out) -> Merge/1
  decrease temperature/1(temperature_out) -> Merge/2
  Crank deserialize event1/2 -> decrease temperature/1(num)
  Crank deserialize event1/1 -> decrease temperature/Trigger
  Crank deserialize event/1 -> Increase temperature/Trigger
  Crank deserialize event/2 -> Increase temperature/1(num)
  event/1 -> Crank deserialize event/1, Crank deserialize event1/1, Crank deserialize event2/1, Crank deserialize event3/1, Crank deserialize event4/1, Crank deserialize event5/1

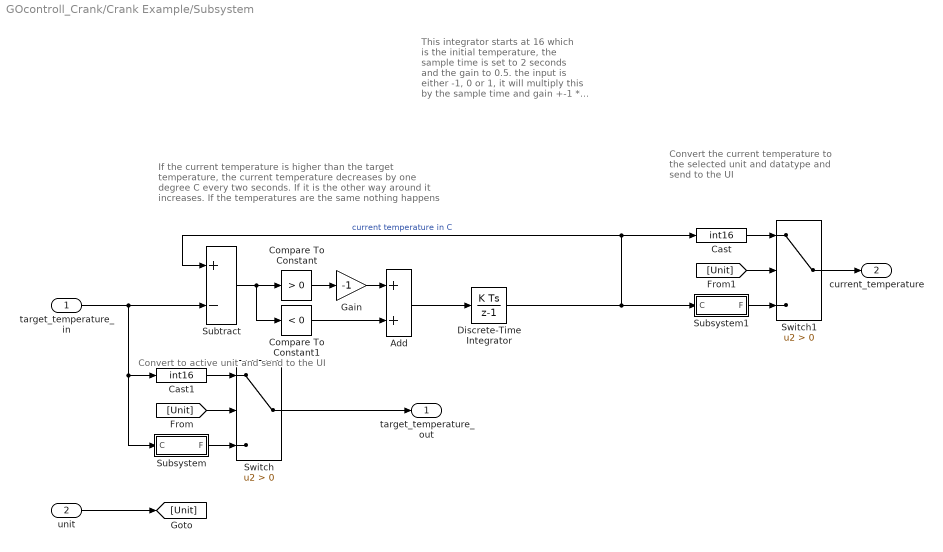
== system GOcontroll_Crank/Crank Example/Subsystem ==
  note: Convert to active unit and send to the UI
  note: If the current temperature is higher than the
      | target temperature, the current temperature
      | decreases by one degree C every two seconds.
      | If it is the other way around it increases. If the
      | temperatures are the same nothing happens
  note: This integrator starts at
      | 16 which is the initial
      | temperature, the sample
      | time is set to 2 seconds
      | and the gain to 0.5.
      | the input is either -1, 0 or
      | 1, it will multiply this by
      | the sample time and gain
      | +-1 * 2 *0.5 is +-1 again.
      | The sample time could be
      | made faster to update the
      | UI faster, especially in the
      | case of fahrenheit this
      | might look better
  note: Convert the current
      | temperature to the selected
      | unit and datatype and send
      | to the UI
  target_temperature_in : Inport
  unit : Inport  Port=2
  Add : Sum  OutDataTypeStr=int16  AccumDataTypeStr=int16
  Cast : DataTypeConversion  OutDataTypeStr=int16  SaturateOnIntegerOverflow=off  RndMeth=Floor
  Cast1 : DataTypeConversion  OutDataTypeStr=int16  SaturateOnIntegerOverflow=off  RndMeth=Floor
  Compare To Constant : simulink/Logic and Bit Operations/Compare To Constant  relop=>  const=0  OutDataTypeStr=uint8
  Compare To Constant1 : simulink/Logic and Bit Operations/Compare To Constant  relop=<  const=0  OutDataTypeStr=uint8
  Discrete-Time Integrator : DiscreteIntegrator  gainval=0.5  InitialCondition=16  SampleTime=2  OutDataTypeStr=single  ICPrevOutput=DiscIntNeverNeededParam  ICPrevScaledInput=DiscIntNeverNeededParam
  Gain : Gain  Gain=-1  ParamDataTypeStr=int16  OutDataTypeStr=single
  Subsystem : Subsystem
  Subsystem1 : Subsystem
  Subtract : Sum  Inputs=+-
  Switch : Switch  Criteria=u2 > Threshold  SaturateOnIntegerOverflow=off  InputSameDT=off
  Switch1 : Switch  Criteria=u2 > Threshold  SaturateOnIntegerOverflow=off  InputSameDT=off
  target_temperature_out : Outport
  current_temperature : Outport  Port=2
  wires:
  Cast1/1 -> Switch/1
  Cast/1 -> Switch1/1
  Switch1/1 -> current_temperature/1
  Subsystem1/1(F) -> Switch1/3
  Discrete-Time Integrator/1 -> Cast/1, Subtract/1, Subsystem1/1(C)  "current temperature in C"
  [Unit] -> Switch1/2
  unit/1 -> [Unit]
  [Unit] -> Switch/2
  target_temperature_in/1 -> Subtract/2, Cast1/1, Subsystem/1(C)
  Subsystem/1(F) -> Switch/3
  Switch/1 -> target_temperature_out/1
  Add/1 -> Discrete-Time Integrator/1
  Compare To Constant1/1 -> Add/2
  Gain/1 -> Add/1
  Compare To Constant/1 -> Gain/1
  Subtract/1 -> Compare To Constant/1, Compare To Constant1/1

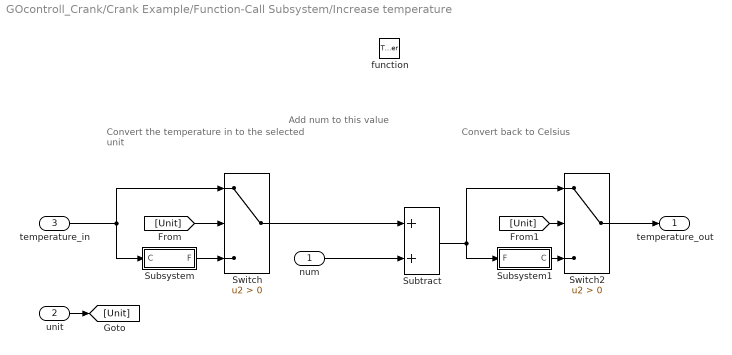
== system GOcontroll_Crank/Crank Example/Function-Call Subsystem/Increase temperature ==
  note: Convert the temperature in to
      | the selected unit
  note: Add num to this value
  note: Convert back to Celsius
  num : Inport
  unit : Inport  Port=2
  temperature_in : Inport  Port=3  Unit=degC
  function : TriggerPort  TriggerType=function-call  VariantControl=(inherit)
  Subsystem : Subsystem
  Subsystem1 : Subsystem
  Subtract : Sum  OutDataTypeStr=single  AccumDataTypeStr=single
  Switch : Switch  Criteria=u2 > Threshold  SaturateOnIntegerOverflow=off  InputSameDT=off
  Switch2 : Switch  Criteria=u2 > Threshold  SaturateOnIntegerOverflow=off  InputSameDT=off
  temperature_out : Outport  InitialOutput=single(16)
  wires:
  Subsystem1/1(C) -> Switch2/3
  temperature_in/1 -> Switch/1, Subsystem/1(C)
  Subsystem/1(F) -> Switch/3
  Switch2/1 -> temperature_out/1
  Subtract/1 -> Subsystem1/1(F), Switch2/1
  [Unit] -> Switch2/2
  unit/1 -> [Unit]
  [Unit] -> Switch/2
  num/1 -> Subtract/2
  Switch/1 -> Subtract/1
